simulink model "deltasigma3"  (Simulink 7.6)
settings: Solver=ode45  StartTime=0.0  StopTime=2  MaxStep=5/1024  RelTol=1e-3
libraries: simeventssignalmanage1 x4, dsparch4 x1, simulink_extras x1, simulink x1, dspsrcs4 x1
settings Model: Creator=Robin  LastModifiedBy=Robin
settings SimEventsCC: propDiagAttribOutput=1  propDiagFcnCallOutput=1  propDiagStatOutput=0

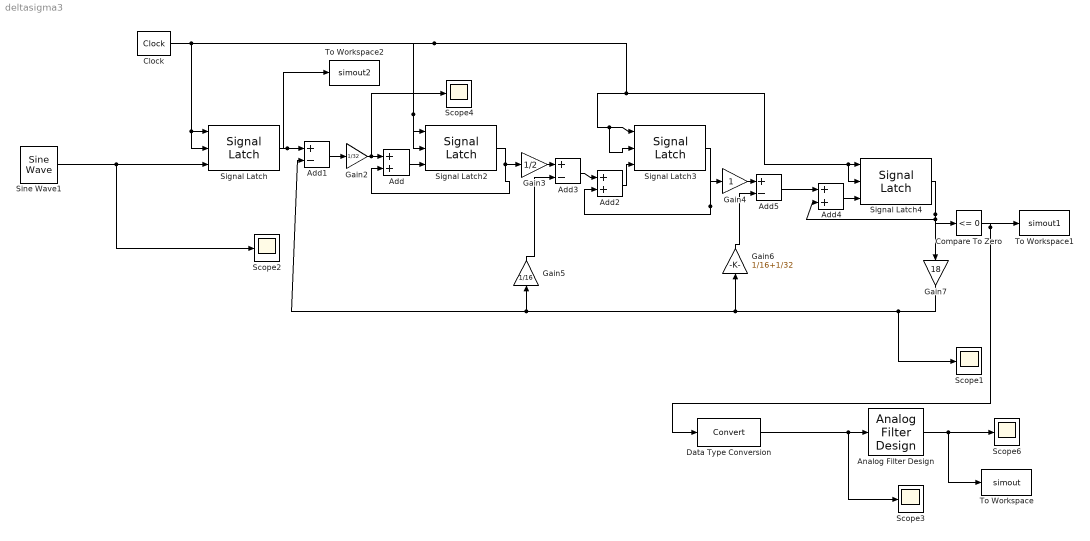
== system deltasigma3 ==
  Add : Sum  AccumDataTypeStr=int16  RndMeth=Convergent
  Add1 : Sum  Inputs=+-  AccumDataTypeStr=int16  RndMeth=Nearest
  Add2 : Sum  AccumDataTypeStr=int16  RndMeth=Convergent
  Add3 : Sum  Inputs=+-  AccumDataTypeStr=int16  RndMeth=Convergent
  Add4 : Sum  AccumDataTypeStr=int16  RndMeth=Convergent
  Add5 : Sum  Inputs=+-  AccumDataTypeStr=int16  RndMeth=Convergent
  Analog Filter Design : dsparch4/Analog Filter Design  method=Butterworth  filttype=Lowpass  N=3  Wlo=2*pi*50  Whi=10*pi  Rp=2  Rs=40
  Clock : simulink_extras/Flip Flops/Clock  SystemSampleTime=-1  period=1/1000
  Compare To Zero : simulink/Logic and Bit Operations/Compare To Zero  SystemSampleTime=-1  relop=<=  LogicOutDataTypeMode=uint8
  Data Type Conversion : DataTypeConversion  RndMeth=Convergent
  Gain2 : Gain  Gain=1/32
  Gain3 : Gain  Gain=1/2
  Gain4 : Gain
  Gain5 : Gain  Gain=1/16
  Gain6 : Gain  Gain=1/16+1/32
  Gain7 : Gain  Gain=18
  Scope{1..4,6} (5 alike) : Scope
      Scope3 settings: TimeRange=1  YMin=-1  YMax=15  SaveName=ScopeData2
      Scope4 settings: SaveName=ScopeData3
      Scope6 settings: TimeRange=1.085543199315655  YMin=-0.2  YMax=0.1776315789473685  SaveName=ScopeData4
  Signal Latch{,2..4} (4 alike) : simeventssignalmanage1/Signal Latch  SystemSampleTime=-1  InitialMemoryValue=0  WriteMemoryUpon=Change in signal from port wvc  MemoryWriteEdgeOption=Rising  SpecifyWriteEventPriority=on  PriorityMemoryWrite=7100  ReadMemoryUpon=Change in signal from port rvc  MemoryReadEdgeOption=Falling  SpecifyReadEventPriority=on  PriorityMemoryRead=7000  ReportMemoryState=off  ReportMemoryUponWrite=off  ReportMemoryUponRead=on
  Sine Wave1 : dspsrcs4/Sine Wave  Amplitude=2^12  Frequency=40  Phase=0  SampleMode=Discrete  OutComplex=Real  CompMethod=Trigonometric fcn  TableSize=Speed  SampleTime=1/1024  SamplesPerFrame=1  ResetState=Restart at time zero  dataType=double  wordLen=16  udDataType=sfix(16)  fracBitsMode=Best precision  numFracBits=15  OutDataTypeStr=double  LastOutDataTypeStr=double
  To Workspace : ToWorkspace  VariableName=simout  SampleTime=-1  SaveFormat=Structure With Time
  To Workspace1 : ToWorkspace  VariableName=simout1  SampleTime=-1  SaveFormat=Structure With Time
  To Workspace2 : ToWorkspace  VariableName=simout2  SampleTime=-1  SaveFormat=Structure With Time
  wires:
  Signal Latch/1 -> Add1/1, To Workspace2/1
  Add3/1 -> Add2/1
  Add1/1 -> Gain2/1
  Data Type Conversion/1 -> Analog Filter Design/1, Scope3/1
  Add/1 -> Signal Latch2/3
  Signal Latch2/1 -> Add/2, Gain3/1
  Add2/1 -> Signal Latch3/3
  Signal Latch3/1 -> Add2/2, Gain4/1
  Add5/1 -> Add4/1
  Add4/1 -> Signal Latch4/3
  Signal Latch4/1 -> Compare To Zero/1, Add4/2, Gain7/1
  Clock/1 -> Signal Latch/1, Signal Latch/2, Signal Latch2/1, Signal Latch2/2, Signal Latch3/1, Signal Latch3/2, Signal Latch4/1, Signal Latch4/2
  Gain2/1 -> Add/1, Scope4/1
  Gain3/1 -> Add3/1
  Gain4/1 -> Add5/1
  Gain6/1 -> Add5/2
  Gain5/1 -> Add3/2
  Gain7/1 -> Scope1/1, Add1/2, Gain5/1, Gain6/1
  Analog Filter Design/1 -> To Workspace/1, Scope6/1
  Compare To Zero/1 -> Data Type Conversion/1, To Workspace1/1
  Sine Wave1/1 -> Scope2/1, Signal Latch/3
